simulink model "ComparisonDinamiche"  (R2020b)
settings: Solver=VariableStepAuto  StartTime=0.0  StopTime=5  RelTol=1e-3
values from neighbouring files (symbols this model uses):
  A_num = eval(A)    [eq_non_linear.m]
  B_num = eval(B)    [eq_non_linear.m]
  C_num = eval(C)    [eq_non_linear.m]
  D_num = eval(D)    [eq_non_linear.m]
  reg_dir_R = ss(A_R-B_R*K_R-L_R*C_R,L_R,K_R,0)    [controllo.m]
  reg_dir_Y = ss(A_Y-B_Y*K_Y-L_Y*C_Y,L_Y,K_Y,0)    [controllo.m]
  reg_dir_z = ss(A_z-B_z*K_z-L_z*C_z,L_z,K_z,0)    [controllo.m]
libraries: pid_lib x1, simulink x1
settings Model: Creator=Tommaso  LastModifiedBy=Tommaso

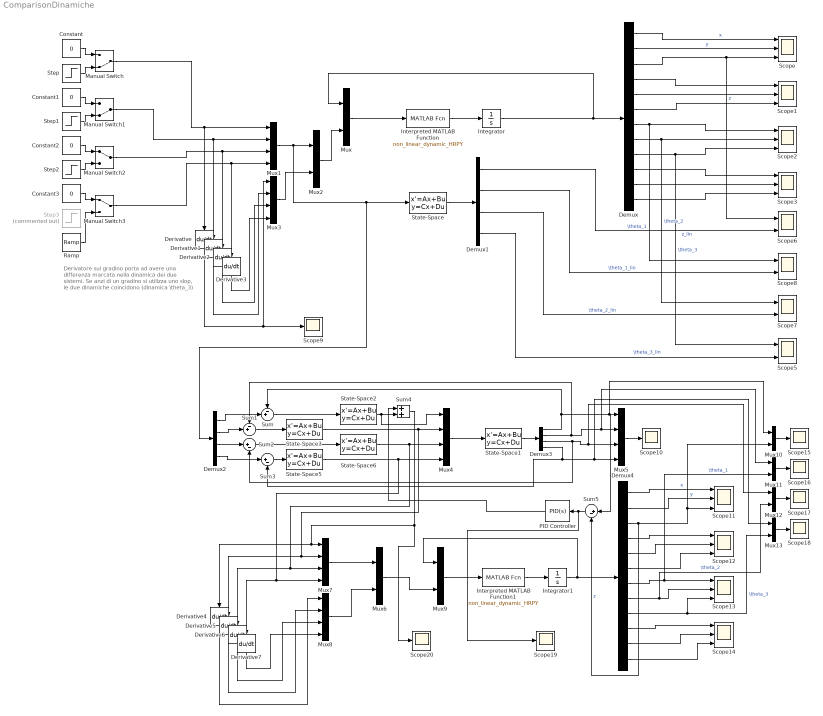
== system ComparisonDinamiche ==
  note: Derivatore sul gradino porta ad avere una differenza
      | marcata nella dinamica dei due sistemi. Se anzi di un gradino
      | si utilizza uno slop, le due dinamiche coincidono
      | (dinamica \theta_3)
  Constant{,1..3} (4 alike) : Constant  Value=0
  Demux : Demux  Outputs=12
  Demux1 : Demux
  Demux2 : Demux
  Demux3 : Demux
  Demux4 : Demux  Outputs=12
  Derivative{,1..7} (8 alike) : Derivative
  Integrator : Integrator  InitialCondition=[0,0,0,0,0,0,0,0,0,0,0,0]
  Integrator1 : Integrator  InitialCondition=[0,0,0,0,0,0,0,0,0,0,0,0]
  Interpreted MATLAB Function : MATLABFcn  MATLABFcn=non_linear_dynamic_HRPY
  Interpreted MATLAB Function1 : MATLABFcn  MATLABFcn=non_linear_dynamic_HRPY
  Manual Switch : ManualSwitch  CurrentSetting=0
  Manual Switch1 : ManualSwitch  CurrentSetting=0
  Manual Switch2 : ManualSwitch
  Manual Switch3 : ManualSwitch
  Mux{,2,6,9..13} (8 alike) : Mux  Inputs=2
  Mux{1,3..5,7..8} (6 alike) : Mux
  PID Controller : pid_lib/PID Controller  Controller=PID  Form=Parallel  TimeDomain=Continuous-time  UseExternalTs=off  SampleTime=-1  IntegratorMethod=Forward Euler  FilterMethod=Forward Euler  ControllerParametersSource=internal  P=1  I=0.4  D=0.8  UseFilter=on  N=100  TunerSelectOption=Transfer Function Based (PID Tuner App)  InitialConditionSource=internal  InitialConditionForIntegrator=0  InitialConditionForFilter=0  DifferentiatorICPrevScaledInput=0  ExternalReset=none  TrackingMode=off  Kt=1  LimitOutput=off  SatLimitsSource=internal  UpperSaturationLimit=inf  LowerSaturationLimit=-inf  LinearizeAsGain=on  AntiWindupMode=none  Kb=1  POutMin=[]  POutMax=[]  IOutMin=[]  IOutMax=[]  DOutMin=[]  DOutMax=[]  NOutMin=[]  NOutMax=[]  SumOutMin=[]  SumOutMax=[]  SaturationOutMin=[]  SaturationOutMax=[]  PParamMin=[]  PParamMax=[]  IParamMin=[]  IParamMax=[]  DParamMin=[]  DParamMax=[]  NParamMin=[]  NParamMax=[]  KbParamMin=[]  KbParamMax=[]  KtParamMin=[]  KtParamMax=[]  KbOutMin=[]  KbOutMax=[]  KtOutMin=[]  KtOutMax=[]  IntegratorOutMin=[]  IntegratorOutMax=[]  FilterOutMin=[]  FilterOutMax=[]  SumI1OutMin=[]  SumI1OutMax=[]  SumI2OutMin=[]  SumI2OutMax=[]  SumI3OutMin=[]  SumI3OutMax=[]  SumI4OutMin=[]  SumI4OutMax=[]  SumDOutMin=[]  SumDOutMax=[]  DifferentiatorOutMin=[]  DifferentiatorOutMax=[]  FilterDiffOutCoefMin=[]  FilterDiffOutCoefMax=[]  ReciprocalOutMin=[]  ReciprocalOutMax=[]  SumDenOutMin=[]  SumDenOutMax=[]  SumNumOutMin=[]  SumNumOutMax=[]  DivideOutMin=[]  DivideOutMax=[]  UdiffTsProdOutMin=[]  UdiffTsProdOutMax=[]  NTsProdOutMin=[]  NTsProdOutMax=[]  UintegralTsProdOutMin=[]  UintegralTsProdOutMax=[]  UngainTsProdOutMin=[]  UngainTsProdOutMax=[]  IntegratorContinuousStateAttributes=''  IntegratorStateMustResolveToSignalObject=off  IntegratorRTWStateStorageClass=Auto  FilterContinuousStateAttributes=''  FilterStateMustResolveToSignalObject=off  FilterRTWStateStorageClass=Auto  ParallelPVariant=InternalParameters  IdealPVariant=Disabled  IVariant=InternalParameters  DVariant=InternalParameters  IntegratorVariant=Continuous  SatVariant=Disabled  AWVariant=Passthrough  PCopyVariant=Disabled  TRVariant=Disabled  FdbkBlocksVariant=Forward  IdealPFdbkVariant=Disabled  SatFdbkVariant=Disabled  DerivativeFilterVariant=ContFilter  NVariant=InternalParameters  NCopyVariant=Disabled  FilterICVariant=InternalICsFilter  IntegratorICVariant=InternalICs  ExternalResetVariant=Disabled  TRSumVariant=Passthrough  SumFdbkVariant=Disabled  SumVariant=Sum_PID  TsampFilterVariant=InternalTs  TsampNgainVariant=Passthrough  TsampIntegralVariant=Passthrough  ExternalSaturationOutDataTypeStr=Inherit: Same as second input
  Ramp : simulink/Sources/Ramp  slope=1  start=1  InitialOutput=0
  Scope{,1..3,11..14} (8 alike) : Scope  NumInputPorts=3
  Scope{9..10,15..20} (8 alike) : Scope
  Scope{5..8} (4 alike) : Scope  NumInputPorts=2
  State-Space : StateSpace  A=A_num  B=B_num  C=C_num  D=D_num  InitialCondition=0
  State-Space1 : StateSpace  A=A_num  B=B_num  C=C_num  D=D_num  InitialCondition=0
  State-Space2 : StateSpace  A=reg_dir_z.a  B=reg_dir_z.b  C=reg_dir_z.c  D=reg_dir_z.d  InitialCondition=0
  State-Space3 : StateSpace  A=reg_dir_R.a  B=reg_dir_R.b  C=reg_dir_R.c  D=reg_dir_R.d  InitialCondition=0
  State-Space5 : StateSpace  A=reg_dir_Y.a  B=reg_dir_Y.b  C=reg_dir_Y.c  D=reg_dir_Y.d  InitialCondition=0
  State-Space6 : StateSpace  A=reg_dir_R.a  B=reg_dir_R.b  C=reg_dir_R.c  D=reg_dir_R.d  InitialCondition=0
  Step : Step  SampleTime=0
  Step1 : Step  After=0.1  SampleTime=0
  Step2 : Step  After=0.1  SampleTime=0
  Step3 : Step  Commented=on  After=0.1  SampleTime=0
  Sum : Sum  Inputs=-+|
  Sum1 : Sum  Inputs=-+|
  Sum2 : Sum  Inputs=|+-
  Sum3 : Sum  Inputs=|+-
  Sum4 : Sum
  Sum5 : Sum  Inputs=|+-
  wires:
  Demux/7 -> Scope2/1, Scope8/1  "\\theta_1"
  Interpreted MATLAB Function/1 -> Integrator/1
  Integrator/1 -> Demux/1, Mux/1
  Demux/9 -> Scope2/3, Scope5/1  "\\theta_3"
  Demux/3 -> Scope6/1, Scope/3  "z"
  Demux/2 -> Scope/2  "y"
  Demux/11 -> Scope3/2
  Demux/1 -> Scope/1  "x"
  Demux/10 -> Scope3/1
  Demux/12 -> Scope3/3
  Demux/6 -> Scope1/3
  Mux/1 -> Interpreted MATLAB Function/1
  Demux/5 -> Scope1/2
  Demux/4 -> Scope1/1
  Demux/8 -> Scope2/2, Scope7/1  "\\theta_2"
  Constant/1 -> Manual Switch/1
  Step/1 -> Manual Switch/2
  Manual Switch/1 -> Mux1/1, Derivative/1
  Constant1/1 -> Manual Switch1/1
  Step1/1 -> Manual Switch1/2
  Constant2/1 -> Manual Switch2/1
  Step2/1 -> Manual Switch2/2
  Constant3/1 -> Manual Switch3/1
  Manual Switch1/1 -> Derivative1/1, Mux1/2
  Manual Switch2/1 -> Derivative2/1, Mux1/3
  Manual Switch3/1 -> Derivative3/1, Mux1/4
  Derivative/1 -> Scope9/1, Mux3/1
  Derivative1/1 -> Mux3/2
  Derivative2/1 -> Mux3/3
  Derivative3/1 -> Mux3/4
  Mux2/1 -> Mux/2
  Mux3/1 -> Mux2/2
  State-Space/1 -> Demux1/1
  Demux1/1 -> Scope6/2  "z_lin"
  Demux1/2 -> Scope8/2  "\\theta_1_lin"
  Demux1/3 -> Scope7/2  "\\theta_2_lin"
  Demux1/4 -> Scope5/2  "\\theta_3_lin"
  Ramp/1 -> Manual Switch3/2
  Sum4/1 -> Scope20/1, Derivative4/1, Mux7/1
  Interpreted MATLAB Function1/1 -> Integrator1/1
  Derivative6/1 -> Mux8/3
  Demux4/6 -> Scope12/3
  Sum5/1 -> Scope19/1, PID Controller/1
  Demux3/3 -> Sum2/2, Mux5/3, Mux12/1
  Demux4/9 -> Mux13/2, Scope13/3  "\\theta_3"
  Demux4/10 -> Scope14/1
  Demux2/4 -> Sum3/1
  PID Controller/1 -> Sum4/1
  Mux9/1 -> Interpreted MATLAB Function1/1
  Sum2/1 -> State-Space6/1
  Mux12/1 -> Scope17/1
  Mux13/1 -> Scope18/1
  Mux8/1 -> Mux6/2
  Demux4/7 -> Mux11/2, Scope13/1  "\\theta_1"
  Mux11/1 -> Scope16/1
  Mux10/1 -> Scope15/1
  Derivative4/1 -> Mux8/1
  Derivative5/1 -> Mux8/2
  Mux6/1 -> Mux9/2
  Demux4/2 -> Scope11/2  "y"
  Integrator1/1 -> Mux9/1, Demux4/1
  Demux4/8 -> Mux12/2, Scope13/2  "\\theta_2"
  Demux4/5 -> Scope12/2
  State-Space5/1 -> Mux7/4, Derivative7/1, Mux4/4
  Sum1/1 -> State-Space3/1
  Demux4/3 -> Mux10/2, Scope11/3, Sum5/2  "z"
  Sum3/1 -> State-Space5/1
  Sum/1 -> State-Space2/1
  Mux1/1 -> State-Space/1, Demux2/1, Mux2/1
  Mux4/1 -> State-Space1/1
  Demux2/3 -> Sum2/1
  State-Space6/1 -> Mux7/3, Derivative6/1, Mux4/3
  Derivative7/1 -> Mux8/4
  Mux7/1 -> Mux6/1
  Demux4/1 -> Scope11/1  "x"
  Demux2/1 -> Sum/2
  Demux4/11 -> Scope14/2
  Demux3/1 -> Sum/1, Sum5/1, Mux10/1, Mux5/1
  Demux4/4 -> Scope12/1
  State-Space2/1 -> Mux4/1, Sum4/2
  Demux4/12 -> Scope14/3
  Mux5/1 -> Scope10/1
  Demux2/2 -> Sum1/2
  State-Space3/1 -> Derivative5/1, Mux7/2, Mux4/2
  Demux3/4 -> Mux5/4, Mux13/1, Sum3/2
  State-Space1/1 -> Demux3/1
  Demux3/2 -> Mux5/2, Mux11/1, Sum1/1
